simulink model "tisch"  (R2015a)
settings: Solver=ode45  StartTime=0.0  StopTime=10  RelTol=1e-3
settings Model: Creator=abg687  LastModifiedBy=leon
settings DebuggingCC: UnderspecifiedInitializationDetection=Classic  MergeDetectMultiDrivingBlocksExec=none  SolverPrmCheckMsg=warning

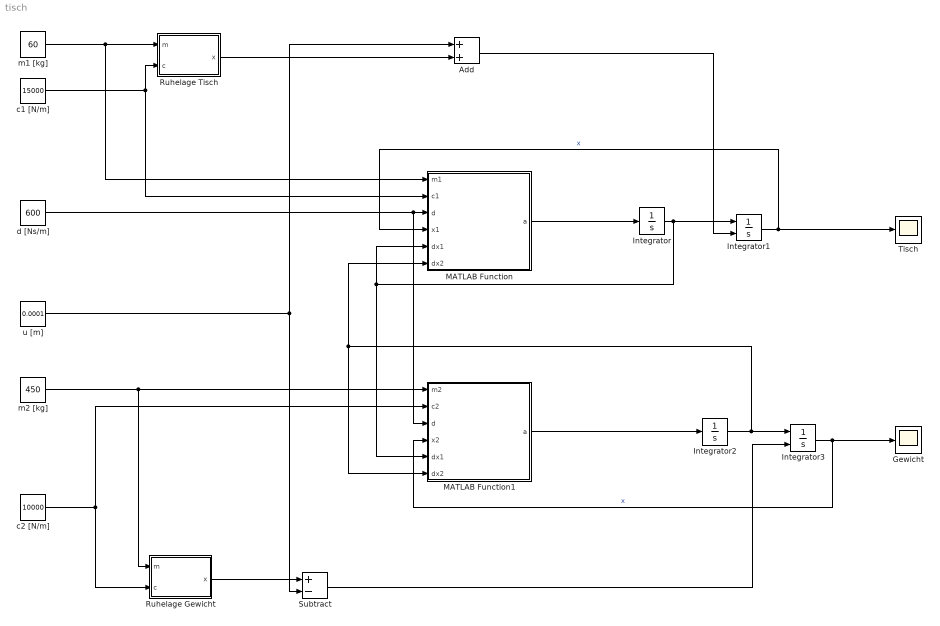
== system tisch ==
  Add : Sum
  Gewicht : Scope
  Integrator : Integrator
  Integrator1 : Integrator  InitialConditionSource=external
  Integrator2 : Integrator
  Integrator3 : Integrator  InitialConditionSource=external
  MATLAB Function : MATLAB Function  TreatAsAtomicUnit=on
  MATLAB Function1 : MATLAB Function  TreatAsAtomicUnit=on
  Ruhelage Gewicht : MATLAB Function  TreatAsAtomicUnit=on
  Ruhelage Tisch : MATLAB Function  TreatAsAtomicUnit=on
  Subtract : Sum  Inputs=+-
  Tisch : Scope
  c1 [N/m] : Constant  Value=15000
  c2 [N/m] : Constant  Value=10000
  d [Ns/m] : Constant  Value=600
  m1 [kg] : Constant  Value=60
  m2 [kg] : Constant  Value=450
  u [m] : Constant  Value=0.0001
  wires:
  m1 [kg]/1 -> MATLAB Function/1(m1), Ruhelage Tisch/1(m)
  c1 [N/m]/1 -> MATLAB Function/2(c1), Ruhelage Tisch/2(c)
  u [m]/1 -> Add/1, Subtract/2
  Add/1 -> Integrator1/2
  d [Ns/m]/1 -> MATLAB Function1/3(d), MATLAB Function/3(d)
  Ruhelage Tisch/1(x) -> Add/2
  MATLAB Function/1(a) -> Integrator/1
  Integrator/1 -> MATLAB Function/5(dx1), MATLAB Function1/5(dx1), Integrator1/1
  Integrator1/1 -> Tisch/1, MATLAB Function/4(x1)  "x"
  m2 [kg]/1 -> MATLAB Function1/1(m2), Ruhelage Gewicht/1(m)
  c2 [N/m]/1 -> MATLAB Function1/2(c2), Ruhelage Gewicht/2(c)
  Ruhelage Gewicht/1(x) -> Subtract/1
  MATLAB Function1/1(a) -> Integrator2/1
  Subtract/1 -> Integrator3/2
  Integrator2/1 -> MATLAB Function/6(dx2), MATLAB Function1/6(dx2), Integrator3/1
  Integrator3/1 -> MATLAB Function1/4(x2), Gewicht/1  "x"

== matlab function tisch/MATLAB Function ==
  data: m1 input; a output; c1 input; d input; x1 input; dx1 input; dx2 input
function a = fcn(m1,c1,d,x1,dx1, dx2)
g = 9.81;

%Federkraft
FF = -c1 * x1;

%Dämpfung
FD = d * (dx1 - dx2);

a = ((2*FF - 2*FD)/m1) -g;

== matlab function tisch/Ruhelage Tisch ==
  data: m input; x output; c input
function x = fcn(m, c)
g = 9.81;
x = (m*g)/(2*c);

== matlab function tisch/Ruhelage Gewicht ==
  data: m input; x output; c input
function x = fcn(m, c)
g = 9.81;
x = (m*g)/(2*c);

== matlab function tisch/MATLAB Function1 ==
  data: m2 input; a output; c2 input; d input; x2 input; dx1 input; dx2 input
function a = fcn(m2,c2,d,x2,dx1, dx2)
g = 9.81;
%Federkraft
FF = -c2 * x2;

%Dämpfung
FD = d * (dx1 - dx2);

a = ((2 * FF + 2 * FD) / m2) - g;
